simulink model "PV_model"  (R2018b)
settings: Solver=ode15s  StartTime=0.0  StopTime=6300  MaxStep=0.4  RelTol=1e-3  EnableMultiTasking=on
InitFcn:
  | load model_data
StopFcn:
  | %Title: System Identification for a HVAC Model
  | %Authors: Harsha Mathur and Nassim Khaled
  | %Last Modified: 4/11/2019
  | 
  | %% Plotting Settings
  | set(0,'DefaultLineLineWidth',2)
  | set(0,'DefaultAxesFontWeight','bold')
  | set(0,'DefaultAxesFontName','Arial')
  | set(0,'DefaultAxesFontSize',12)
  | 
  | figure
  | subplot(2,1,1)
  | 
  | plot(Time_sim,Voltage_PV1_measured)
  | hold on
  | plot(Time_sim,Voltage_PV1_sim,'r')
  | title('PV 1')
  | legend('Measured','simulated')
  | ylabel('Voltage [V]')
  | ylim([0 15])
  | grid on
  | 
  | subplot(2,1,2)
  | plot(Time_sim,Power_PV1_measured)
  | hold on
  | plot(Time_sim,Power_PV1_sim,'r')
  | legend('Measured','simulated')
  | ylabel('Power [Watts]')
  | ylim([0 100])
  | grid on
  | xlabel('Time [sec]')
  | 
  | 
  | figure
  | subplot(2,1,1)
  | 
  | plot(Time_sim,Voltage_PV23_measured)
  | hold on
  | plot(Time_sim,Voltage_PV23_sim,'r')
  | title('PV 2 and 3')
  | legend('Measured','simulated')
  | ylabel('Voltage [V]')
  | ylim([0 15])
  | grid on
  | 
  | subplot(2,1,2)
  | plot(Time_sim,Power_PV23_measured)
  | hold on
  | plot(Time_sim,Power_PV23_sim,'r')
  | legend('Measured','simulated')
  | ylabel('Power [Watts]')
  | ylim([0 100])
  | grid on
  | xlabel('Time [sec]')
undefined symbols (not defined in the file or in its folder): C1_LUT, Capacity_LUT, cell_Cp_heat, cell_mass, Em_LUT, Qe_init, R0_LUT, R1_LUT, SOC_LUT, T_init, Temperature_LUT
libraries: elec_lib x117, fl_lib x36, LiBatteryElements_lib x12, nesl_utility x12
settings Model: Creator=Sanjay Lodwal  LastModifiedBy=user
settings DataIOCC: LimitDataPoints=on  SaveFormat=Array
settings OptimizationCC: LifeSpan=inf
settings DebuggingCC: UnderspecifiedInitializationDetection=Classic  MergeDetectMultiDrivingBlocksExec=none  SolverPrmCheckMsg=warning  StateNameClashWarn=warning  SFUnexpectedBacktrackingDiag=warning  SFNoUnconditionalDefaultTransitionDiag=warning  SFExecutionAtInitializationDiag=none
settings HardwareCC: ProdBitPerPointer=32  ProdBitPerSizeT=32  ProdBitPerPtrDiffT=32  ProdLargestAtomicFloat=None  ProdIntDivRoundTo=Undefined  ProdEndianess=Unspecified  ProdWordSize=32  ProdHWDeviceType=32-bit Generic
settings ModelReferenceCC: PropagateSignalLabelsOutOfModel=off
settings SFSimCC: SimUseLocalCustomCode=off
settings RTWCC: RTWUseLocalCustomCode=off
settings CodeAppCC: StateflowObjectComments=on
settings GRTTargetCC: TargetLangStandard=C89/C90 (ANSI)  GeneratePreprocessorConditionals=Disable all
settings ConfigComp: CovMetricSettings=dw  CovHtmlReporting=on  CovSaveCumulativeToWorkspaceVar=on  CovSaveSingleToWorkspaceVar=on  CovExternalEMLEnable=off
settings SimscapeCC: SimscapeNormalizeSystem=off

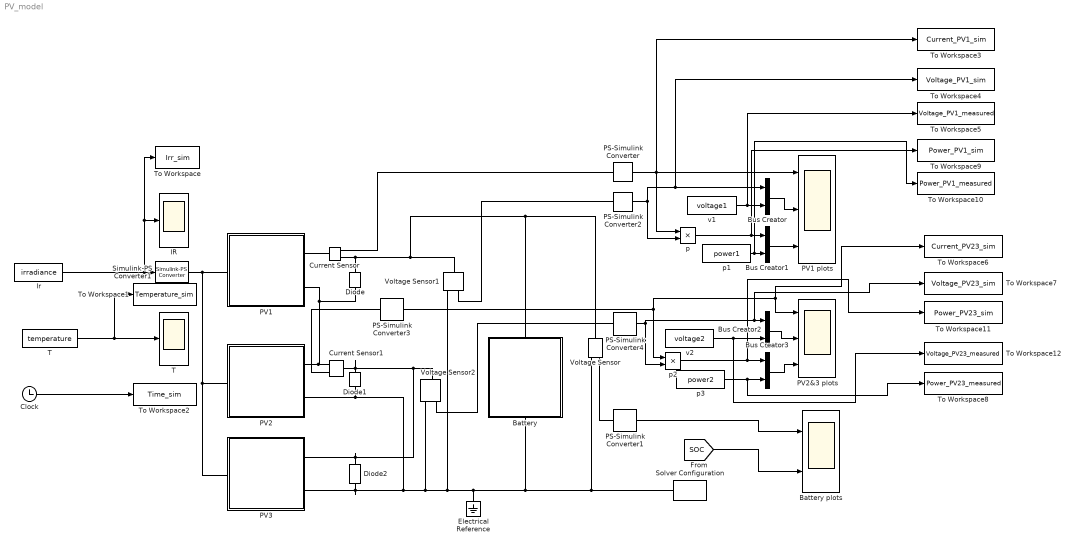
== system PV_model ==
  "\tT" : Scope
  Battery : Subsystem
      mask Display: image('battery.png')
  Battery plots : Scope  NumInputPorts=2
  Bus Creator{,1..3} (4 alike) : BusCreator  Inputs=2
  Clock : Clock
  Current Sensor : fl_lib/Electrical/Electrical Sensors/Current Sensor
  Current Sensor1 : fl_lib/Electrical/Electrical Sensors/Current Sensor
  Diode : fl_lib/Electrical/Electrical Elements/Diode  Vf=0.6 V  Ron=0.3 Ohm  Goff=1e-8 1/Ohm  i_specify=off  i_priority=High  i=0 A  i_nominal_specify=off  i_nominal_unit=A  i_nominal_value=1  v_specify=off  v_priority=High  v=0 V  v_nominal_specify=off  v_nominal_unit=V  v_nominal_value=1
  Diode1 : fl_lib/Electrical/Electrical Elements/Diode  Vf=0.6 V  Ron=0.3 Ohm  Goff=1e-8 1/Ohm  i_specify=off  i_priority=High  i=0 A  i_nominal_specify=off  i_nominal_unit=A  i_nominal_value=1  v_specify=off  v_priority=High  v=0 V  v_nominal_specify=off  v_nominal_unit=V  v_nominal_value=1
  Diode2 : fl_lib/Electrical/Electrical Elements/Diode  Vf=0.6 V  Ron=0.3 Ohm  Goff=1e-8 1/Ohm  i_specify=off  i_priority=High  i=0 A  i_nominal_specify=off  i_nominal_unit=A  i_nominal_value=1  v_specify=off  v_priority=High  v=0 V  v_nominal_specify=off  v_nominal_unit=V  v_nominal_value=1
  Electrical Reference : fl_lib/Electrical/Electrical Elements/Electrical Reference
  IR : Scope
  Ir : FromWorkspace  VariableName=irradiance  SampleTime=0
  PS-Simulink Converter{,1..4} (5 alike) : nesl_utility/PS-Simulink Converter  PhysicalDomain=network_engine_domain  SubClassName=ps_output  LeftPortType=input  RightPortType=output  PseudoPeriodic=off  Frequencies=[]  Unit=1  AffineConversion=off
  PV1 : Subsystem  mask{Isc=5.49, Voc=21.5, n=1.5, Rs=0, Ir0=1000, T=30}
      mask prompts: Isc "Short circuit current"; Voc "Open circuit voltage"; n "Quality factor, N"; Rs "Series resistance"; Ir0 "Reference irradiation"; T "Temperature"
      mask Display: image('PV1.jpg')
  PV1 plots : Scope  NumInputPorts=3
  PV2 : Subsystem  mask{Isc=6.37, Voc=21.5, n=1.5, Rs=0, Ir0=1000, T=30}
      mask prompts: Isc "Short circuit current"; Voc "Open circuit voltage"; n "Quality factor, N"; Rs "Series resistance"; Ir0 "Reference irradiation"; T "Temperature"
      mask Display: image('PV2.jpg')
  PV2&3 plots : Scope  NumInputPorts=3
  PV3 : Subsystem  mask{Isc=6.37, Voc=21.5, n=1.5, Rs=0, Ir0=1000, T=30}
      mask prompts: Isc "Short circuit current"; Voc "Open circuit voltage"; n "Quality factor, N"; Rs "Series resistance"; Ir0 "Reference irradiation"; T "Temperature"
      mask Display: image('PV3.jpg')
  Simulink-PS Converter1 : nesl_utility/Simulink-PS Converter  PhysicalDomain=network_engine_domain  SubClassName=ps_input  LeftPortType=input  RightPortType=output  PseudoPeriodic=off  Frequencies=[]  NoiseDistribution=none  NoiseParameters=[]  Unit=1  AffineConversion=off  FilteringAndDerivatives=zero  SimscapeFilterOrder=1  InputFilterTimeConstant=0.001  UdotUserProvided=1
  Solver Configuration : nesl_utility/Solver Configuration  PhysicalDomain=network_engine_domain  SubClassName=solver  LeftPortType=input  RightPortType=generic  Tones=[]  Harmonics=[]  SimulateNoise=off  Profile=off  UseLocalSampling=off  EnableSwitchedLinearOptims=on  FrequencyDomain=off  UseCCode=off  RelTol=0.001  AbsTol=1e-06  MinStep=1e-09  ToWorkspace=off  RevertToSquareIcSolve=off  NumHomotopyIterations=100  PhasorMode=off  PhasorModeNumHarmonics=1  DoDC=off  ResidualTolerance=1e-09  UseLocalSolver=off  LocalSolverChoice=NE_BACKWARD_EULER_ADVANCER  LocalSolverSampleTime=0.001  DoFixedCost=off  MaxNonlinIter=3  MaxModeIter=2  LinearAlgebra=Sparse  EquationFormulation=NE_TIME_EF  DelaysMemoryBudget=1024  AutomaticFiltering=on  FilteringTimeConstant=0.001  PartitionStorageMethod=AS_NEEDED  PartitionMemoryBudget=1024
  T : FromWorkspace  VariableName=temperature  SampleTime=0
  To Workspace : ToWorkspace  VariableName=Irr_sim  SampleTime=-1
  To Workspace1 : ToWorkspace  VariableName=Temperature_sim  SampleTime=-1
  To Workspace10 : ToWorkspace  VariableName=Power_PV1_measured  SampleTime=-1
  To Workspace11 : ToWorkspace  VariableName=Power_PV23_sim  SampleTime=-1
  To Workspace12 : ToWorkspace  VariableName=Voltage_PV23_measured  SampleTime=-1
  To Workspace2 : ToWorkspace  VariableName=Time_sim  SampleTime=-1
  To Workspace3 : ToWorkspace  VariableName=Current_PV1_sim  SampleTime=-1
  To Workspace4 : ToWorkspace  VariableName=Voltage_PV1_sim  SampleTime=-1
  To Workspace5 : ToWorkspace  VariableName=Voltage_PV1_measured  SampleTime=-1
  To Workspace6 : ToWorkspace  VariableName=Current_PV23_sim  SampleTime=-1
  To Workspace7 : ToWorkspace  VariableName=Voltage_PV23_sim  SampleTime=-1
  To Workspace8 : ToWorkspace  VariableName=Power_PV23_measured  SampleTime=-1
  To Workspace9 : ToWorkspace  VariableName=Power_PV1_sim  SampleTime=-1
  Voltage Sensor : fl_lib/Electrical/Electrical Sensors/Voltage Sensor
  Voltage Sensor1 : fl_lib/Electrical/Electrical Sensors/Voltage Sensor
  Voltage Sensor2 : fl_lib/Electrical/Electrical Sensors/Voltage Sensor
  p : Product
  p1 : FromWorkspace  VariableName=power1  SampleTime=0
  p2 : Product
  p3 : FromWorkspace  VariableName=power2  SampleTime=0
  v1 : FromWorkspace  VariableName=voltage1  SampleTime=0
  v2 : FromWorkspace  VariableName=voltage2  SampleTime=0
  wires:
  Ir/1 -> To Workspace/1, IR/1, Simulink-PS Converter1/1
  PS-Simulink Converter/1 -> To Workspace3/1, PV1 plots/1, p/1
  PS-Simulink Converter2/1 -> To Workspace4/1, Bus Creator/1, p/2
  PS-Simulink Converter4/1 -> p2/2, To Workspace7/1, Bus Creator2/1
  [SOC] -> Battery plots/2
  PS-Simulink Converter1/1 -> Battery plots/1
  T/1 -> To Workspace1/1, "\tT"/1
  v1/1 -> To Workspace5/1, Bus Creator/2
  Bus Creator/1 -> PV1 plots/2
  Bus Creator1/1 -> PV1 plots/3
  p/1 -> To Workspace9/1, Bus Creator1/1
  p1/1 -> To Workspace10/1, Bus Creator1/2
  PS-Simulink Converter3/1 -> To Workspace6/1, PV2&3 plots/1, p2/1
  Bus Creator2/1 -> PV2&3 plots/2
  v2/1 -> To Workspace12/1, Bus Creator2/2
  p2/1 -> To Workspace11/1, Bus Creator3/1
  p3/1 -> To Workspace8/1, Bus Creator3/2
  Bus Creator3/1 -> PV2&3 plots/3
  Clock/1 -> To Workspace2/1
  connections:
  Simulink-PS Converter1/RConn1 -- PV3/LConn1 -- PV2/LConn1 -- PV1/LConn1
  Current Sensor/RConn1 -- PS-Simulink Converter/LConn1
  PS-Simulink Converter1/LConn1 -- Voltage Sensor/RConn1
  Battery/RConn1 -- Voltage Sensor/LConn1 -- Voltage Sensor1/LConn1 -- Diode/RConn1 -- Current Sensor/RConn2
  Diode1/RConn1 -- Current Sensor1/LConn1 -- Voltage Sensor2/LConn1 -- PV3/RConn1 -- Diode2/RConn1
  PS-Simulink Converter2/LConn1 -- Voltage Sensor1/RConn1
  PS-Simulink Converter3/LConn1 -- Current Sensor1/RConn1
  PS-Simulink Converter4/LConn1 -- Voltage Sensor2/RConn1
  Solver Configuration/RConn1 -- Battery/LConn1 -- Electrical Reference/LConn1 -- Voltage Sensor1/RConn2 -- PV3/RConn2 -- Diode2/LConn1 -- PV2/RConn2 -- Diode1/LConn1 -- Voltage Sensor2/RConn2 -- Voltage Sensor/RConn2
  Current Sensor/LConn1 -- PV1/RConn1
  PV2/RConn1 -- Diode/LConn1 -- PV1/RConn2 -- Current Sensor1/RConn2

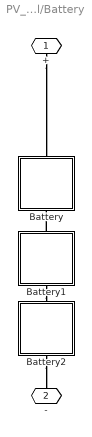
== system PV_model/Battery ==
  Battery : Subsystem  mask(Lithium cell (one RC-branch equivalent circuit)){Qe_init=Qe_init, T_init=T_init, Capacity_LUT=Capacity_LUT, Em_LUT=Em_LUT, R0_LUT=R0_LUT, R1_LUT=R1_LUT, C1_LUT=C1_LUT, cell_mass=cell_mass, cell_Cp_heat=cell_Cp_heat, SOC_LUT=SOC_LUT, Temperature_LUT=Temperature_LUT}
      mask prompts: Qe_init "Initial charge deficit (A*hr)"; T_init "Initial cell temperature (K)"; Capacity_LUT "Capacity (A*hr, 1xN table)"; Em_LUT "Em open-circuit voltage (volts, MxN table)"; R0_LUT "R0 terminal resistance (ohms, MxN table)"; R1_LUT "R1 resistance (ohms, MxN table)"; C1_LUT "C1 capacitance (farads, MxN table)"; cell_mass "Cell mass (kg)"; cell_Cp_heat "Cell specific heat (J/kg/K)"; SOC_LUT "SOC table breakpoints (Mx1 array)"; Temperature_LUT "Temperature table breakpoints (K, 1xN array)"
      mask DialogControl ParameterTabVar0 Prompt: Initial Conditions
      mask DialogControl ParameterTabVar01 Prompt: Electrical
      mask DialogControl ParameterTabVar012 Prompt: Thermal
      mask DialogControl ParameterTabVar0123 Prompt: Table Breakpoints
      mask Display:
      | image('battery.jpg')
      | color('red')
      | port_label('LConn',1,'H')
      | port_label('LConn',2,'+')
      | port_label('RConn',1,'-')
  Battery1 : Subsystem  mask(Lithium cell (one RC-branch equivalent circuit)){Qe_init=Qe_init, T_init=T_init, Capacity_LUT=Capacity_LUT, Em_LUT=Em_LUT, R0_LUT=R0_LUT, R1_LUT=R1_LUT, C1_LUT=C1_LUT, cell_mass=cell_mass, cell_Cp_heat=cell_Cp_heat, SOC_LUT=SOC_LUT, Temperature_LUT=Temperature_LUT}
      mask prompts: Qe_init "Initial charge deficit (A*hr)"; T_init "Initial cell temperature (K)"; Capacity_LUT "Capacity (A*hr, 1xN table)"; Em_LUT "Em open-circuit voltage (volts, MxN table)"; R0_LUT "R0 terminal resistance (ohms, MxN table)"; R1_LUT "R1 resistance (ohms, MxN table)"; C1_LUT "C1 capacitance (farads, MxN table)"; cell_mass "Cell mass (kg)"; cell_Cp_heat "Cell specific heat (J/kg/K)"; SOC_LUT "SOC table breakpoints (Mx1 array)"; Temperature_LUT "Temperature table breakpoints (K, 1xN array)"
      mask DialogControl ParameterTabVar0 Prompt: Initial Conditions
      mask DialogControl ParameterTabVar01 Prompt: Electrical
      mask DialogControl ParameterTabVar012 Prompt: Thermal
      mask DialogControl ParameterTabVar0123 Prompt: Table Breakpoints
      mask Display:
      | image('battery.jpg')
      | color('red')
      | port_label('LConn',1,'H')
      | port_label('LConn',2,'+')
      | port_label('RConn',1,'-')
  Battery2 : Subsystem  mask(Lithium cell (one RC-branch equivalent circuit)){Qe_init=Qe_init, T_init=T_init, Capacity_LUT=Capacity_LUT, Em_LUT=Em_LUT, R0_LUT=R0_LUT, R1_LUT=R1_LUT, C1_LUT=C1_LUT, cell_mass=cell_mass, cell_Cp_heat=cell_Cp_heat, SOC_LUT=SOC_LUT, Temperature_LUT=Temperature_LUT}
      mask prompts: Qe_init "Initial charge deficit (A*hr)"; T_init "Initial cell temperature (K)"; Capacity_LUT "Capacity (A*hr, 1xN table)"; Em_LUT "Em open-circuit voltage (volts, MxN table)"; R0_LUT "R0 terminal resistance (ohms, MxN table)"; R1_LUT "R1 resistance (ohms, MxN table)"; C1_LUT "C1 capacitance (farads, MxN table)"; cell_mass "Cell mass (kg)"; cell_Cp_heat "Cell specific heat (J/kg/K)"; SOC_LUT "SOC table breakpoints (Mx1 array)"; Temperature_LUT "Temperature table breakpoints (K, 1xN array)"
      mask DialogControl ParameterTabVar0 Prompt: Initial Conditions
      mask DialogControl ParameterTabVar01 Prompt: Electrical
      mask DialogControl ParameterTabVar012 Prompt: Thermal
      mask DialogControl ParameterTabVar0123 Prompt: Table Breakpoints
      mask Display:
      | image('battery.jpg')
      | color('red')
      | port_label('LConn',1,'H')
      | port_label('LConn',2,'+')
      | port_label('RConn',1,'-')
  + : PMIOPort  Side=Right
  - : PMIOPort  Port=2  Side=Left
  connections:
  +/RConn1 -- Battery/LConn1
  Battery1/LConn1 -- Battery/RConn1
  Battery1/RConn1 -- Battery2/LConn1
  Battery2/RConn1 -- -/RConn1

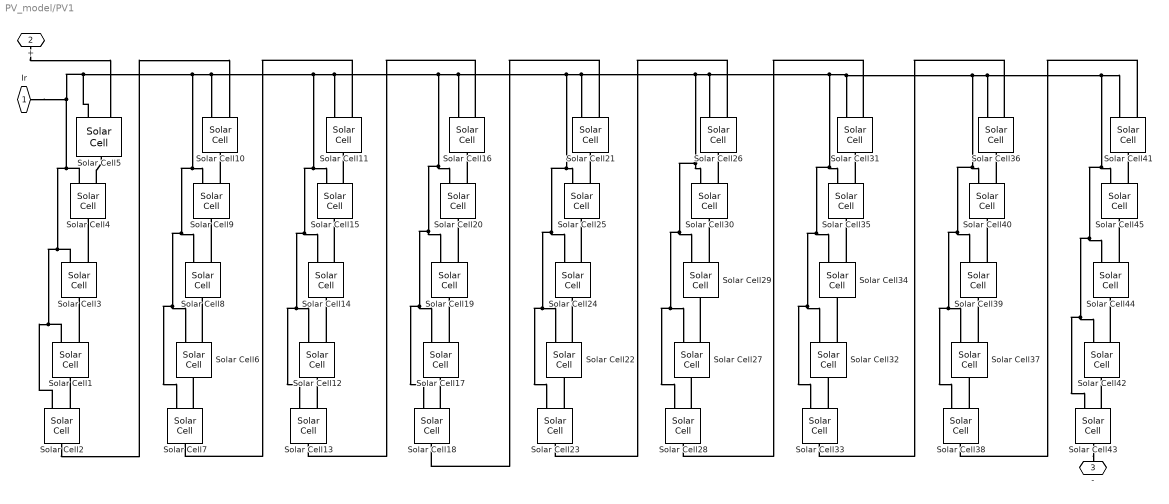
== system PV_model/PV1 ==
  Solar Cell{1..45} (45 alike) : elec_lib/Sources/Solar Cell  prm=1  Isc=Isc A  Voc=Voc/45 V  Is=1e-6 A  Is2=0 A  Iph=7.34 A  Ir0=Ir0 W/m^2  ec=n  N2=2  Rs=Rs/45 Ohm  Rp=Inf Ohm  N_series=1  TIPH1=0 1/K  EG=1.11 eV  TXIS1=3  TXIS2=3  TRS1=0  TRP1=0  Tmeas=T degC  TFIXED=T degC  thermal_mass=100 J/K  initial_temperature=25 degC
      settings: SourceProductName=Simscape Electronics  SourceProductBaseCode=SN
  Ir : PMIOPort  Side=Left
  + : PMIOPort  Port=2  Side=Right
  - : PMIOPort  Port=3  Side=Right
  connections:
  Solar Cell5/LConn1 -- Solar Cell7/LConn1 -- Solar Cell6/LConn1 -- Solar Cell8/LConn1 -- Solar Cell9/LConn1 -- Solar Cell13/LConn1 -- Solar Cell12/LConn1 -- Solar Cell14/LConn1 -- Solar Cell15/LConn1 -- Solar Cell18/LConn1 -- Solar Cell17/LConn1 -- Solar Cell19/LConn1 -- Solar Cell20/LConn1 -- Solar Cell22/LConn1 -- Solar Cell23/LConn1 -- Solar Cell24/LConn1 -- Solar Cell25/LConn1 -- Solar Cell28/LConn1 -- Solar Cell27/LConn1 -- Solar Cell29/LConn1 -- Solar Cell30/LConn1 -- Solar Cell33/LConn1 -- Solar Cell32/LConn1 -- Solar Cell34/LConn1 -- Solar Cell35/LConn1 -- Solar Cell37/LConn1 -- Solar Cell38/LConn1 -- Solar Cell39/LConn1 -- Solar Cell40/LConn1 -- Solar Cell43/LConn1 -- Solar Cell42/LConn1 -- Solar Cell44/LConn1 -- Solar Cell45/LConn1 -- Solar Cell41/LConn1 -- Solar Cell36/LConn1 -- Solar Cell31/LConn1 -- Solar Cell26/LConn1 -- Solar Cell21/LConn1 -- Solar Cell16/LConn1 -- Solar Cell11/LConn1 -- Solar Cell10/LConn1 -- Solar Cell4/LConn1 -- Solar Cell3/LConn1 -- Solar Cell1/LConn1 -- Solar Cell2/LConn1 -- Ir/RConn1
  Solar Cell3/LConn2 -- Solar Cell4/RConn1
  Solar Cell2/LConn2 -- Solar Cell1/RConn1
  Solar Cell1/LConn2 -- Solar Cell3/RConn1
  Solar Cell4/LConn2 -- Solar Cell5/RConn1
  +/RConn1 -- Solar Cell5/LConn2
  Solar Cell9/LConn2 -- Solar Cell10/RConn1
  Solar Cell7/LConn2 -- Solar Cell6/RConn1
  Solar Cell6/LConn2 -- Solar Cell8/RConn1
  Solar Cell2/RConn1 -- Solar Cell10/LConn2
  Solar Cell8/LConn2 -- Solar Cell9/RConn1
  Solar Cell11/LConn2 -- Solar Cell7/RConn1
  Solar Cell12/LConn2 -- Solar Cell14/RConn1
  Solar Cell13/LConn2 -- Solar Cell12/RConn1
  Solar Cell15/LConn2 -- Solar Cell11/RConn1
  Solar Cell14/LConn2 -- Solar Cell15/RConn1
  Solar Cell19/LConn2 -- Solar Cell20/RConn1
  Solar Cell20/LConn2 -- Solar Cell16/RConn1
  Solar Cell16/LConn2 -- Solar Cell13/RConn1
  Solar Cell17/LConn2 -- Solar Cell19/RConn1
  Solar Cell18/LConn2 -- Solar Cell17/RConn1
  Solar Cell23/LConn2 -- Solar Cell22/RConn1
  Solar Cell22/LConn2 -- Solar Cell24/RConn1
  Solar Cell25/LConn2 -- Solar Cell21/RConn1
  Solar Cell21/LConn2 -- Solar Cell18/RConn1
  Solar Cell24/LConn2 -- Solar Cell25/RConn1
  Solar Cell29/LConn2 -- Solar Cell30/RConn1
  Solar Cell26/LConn2 -- Solar Cell23/RConn1
  Solar Cell30/LConn2 -- Solar Cell26/RConn1
  Solar Cell27/LConn2 -- Solar Cell29/RConn1
  Solar Cell28/LConn2 -- Solar Cell27/RConn1
  Solar Cell34/LConn2 -- Solar Cell35/RConn1
  Solar Cell31/LConn2 -- Solar Cell28/RConn1
  Solar Cell35/LConn2 -- Solar Cell31/RConn1
  Solar Cell32/LConn2 -- Solar Cell34/RConn1
  Solar Cell33/LConn2 -- Solar Cell32/RConn1
  Solar Cell39/LConn2 -- Solar Cell40/RConn1
  Solar Cell36/LConn2 -- Solar Cell33/RConn1
  Solar Cell40/LConn2 -- Solar Cell36/RConn1
  Solar Cell37/LConn2 -- Solar Cell39/RConn1
  Solar Cell38/LConn2 -- Solar Cell37/RConn1
  Solar Cell44/LConn2 -- Solar Cell45/RConn1
  Solar Cell41/LConn2 -- Solar Cell38/RConn1
  Solar Cell45/LConn2 -- Solar Cell41/RConn1
  Solar Cell42/LConn2 -- Solar Cell44/RConn1
  Solar Cell43/LConn2 -- Solar Cell42/RConn1
  Solar Cell43/RConn1 -- -/RConn1

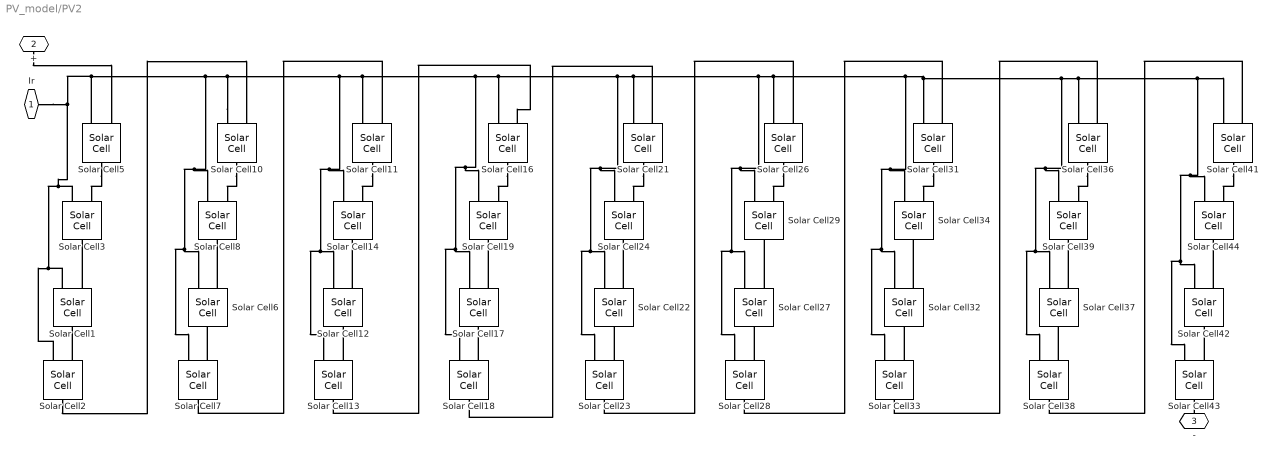
== system PV_model/PV2 ==
  Solar Cell{1..3,5..8,10..14,16..19,21..24,26..29,31..34,36..39,41..44} (36 alike) : elec_lib/Sources/Solar Cell  prm=1  Isc=Isc A  Voc=Voc/45 V  Is=1e-6 A  Is2=0 A  Iph=7.34 A  Ir0=Ir0 W/m^2  ec=n  N2=2  Rs=Rs/45 Ohm  Rp=Inf Ohm  N_series=1  TIPH1=0 1/K  EG=1.11 eV  TXIS1=3  TXIS2=3  TRS1=0  TRP1=0  Tmeas=T degC  TFIXED=T degC  thermal_mass=100 J/K  initial_temperature=25 degC
      settings: SourceProductName=Simscape Electronics  SourceProductBaseCode=SN
  Ir : PMIOPort  Side=Left
  + : PMIOPort  Port=2  Side=Right
  - : PMIOPort  Port=3  Side=Right
  connections:
  Solar Cell10/LConn1 -- Solar Cell13/LConn1 -- Solar Cell12/LConn1 -- Solar Cell14/LConn1 -- Solar Cell18/LConn1 -- Solar Cell17/LConn1 -- Solar Cell19/LConn1 -- Solar Cell22/LConn1 -- Solar Cell23/LConn1 -- Solar Cell24/LConn1 -- Solar Cell28/LConn1 -- Solar Cell27/LConn1 -- Solar Cell29/LConn1 -- Solar Cell33/LConn1 -- Solar Cell32/LConn1 -- Solar Cell34/LConn1 -- Solar Cell37/LConn1 -- Solar Cell38/LConn1 -- Solar Cell39/LConn1 -- Solar Cell41/LConn1 -- Solar Cell43/LConn1 -- Solar Cell42/LConn1 -- Solar Cell44/LConn1 -- Solar Cell36/LConn1 -- Solar Cell31/LConn1 -- Solar Cell26/LConn1 -- Solar Cell21/LConn1 -- Solar Cell16/LConn1 -- Solar Cell11/LConn1 -- Solar Cell5/LConn1 -- Ir/RConn1 -- Solar Cell3/LConn1 -- Solar Cell1/LConn1 -- Solar Cell2/LConn1 -- Solar Cell8/LConn1 -- Solar Cell7/LConn1 -- Solar Cell6/LConn1
  Solar Cell10/RConn1 -- Solar Cell8/LConn2
  Solar Cell1/LConn2 -- Solar Cell3/RConn1
  Solar Cell38/LConn2 -- Solar Cell37/RConn1
  Solar Cell18/LConn2 -- Solar Cell17/RConn1
  Solar Cell7/LConn2 -- Solar Cell6/RConn1
  Solar Cell21/LConn2 -- Solar Cell18/RConn1
  Solar Cell11/RConn1 -- Solar Cell14/LConn2
  Solar Cell31/LConn2 -- Solar Cell28/RConn1
  Solar Cell13/LConn2 -- Solar Cell12/RConn1
  Solar Cell32/LConn2 -- Solar Cell34/RConn1
  Solar Cell22/LConn2 -- Solar Cell24/RConn1
  Solar Cell23/LConn2 -- Solar Cell22/RConn1
  Solar Cell36/LConn2 -- Solar Cell33/RConn1
  Solar Cell2/LConn2 -- Solar Cell1/RConn1
  Solar Cell41/LConn2 -- Solar Cell38/RConn1
  Solar Cell27/LConn2 -- Solar Cell29/RConn1
  Solar Cell12/LConn2 -- Solar Cell14/RConn1
  Solar Cell16/RConn1 -- Solar Cell19/LConn2
  +/RConn1 -- Solar Cell5/LConn2
  Solar Cell28/LConn2 -- Solar Cell27/RConn1
  Solar Cell16/LConn2 -- Solar Cell13/RConn1
  Solar Cell43/LConn2 -- Solar Cell42/RConn1
  Solar Cell33/LConn2 -- Solar Cell32/RConn1
  Solar Cell41/RConn1 -- Solar Cell44/LConn2
  Solar Cell6/LConn2 -- Solar Cell8/RConn1
  Solar Cell2/RConn1 -- Solar Cell10/LConn2
  Solar Cell17/LConn2 -- Solar Cell19/RConn1
  -/RConn1 -- Solar Cell43/RConn1
  Solar Cell11/LConn2 -- Solar Cell7/RConn1
  Solar Cell26/LConn2 -- Solar Cell23/RConn1
  Solar Cell42/LConn2 -- Solar Cell44/RConn1
  Solar Cell37/LConn2 -- Solar Cell39/RConn1
  Solar Cell5/RConn1 -- Solar Cell3/LConn2
  Solar Cell21/RConn1 -- Solar Cell24/LConn2
  Solar Cell26/RConn1 -- Solar Cell29/LConn2
  Solar Cell31/RConn1 -- Solar Cell34/LConn2
  Solar Cell36/RConn1 -- Solar Cell39/LConn2

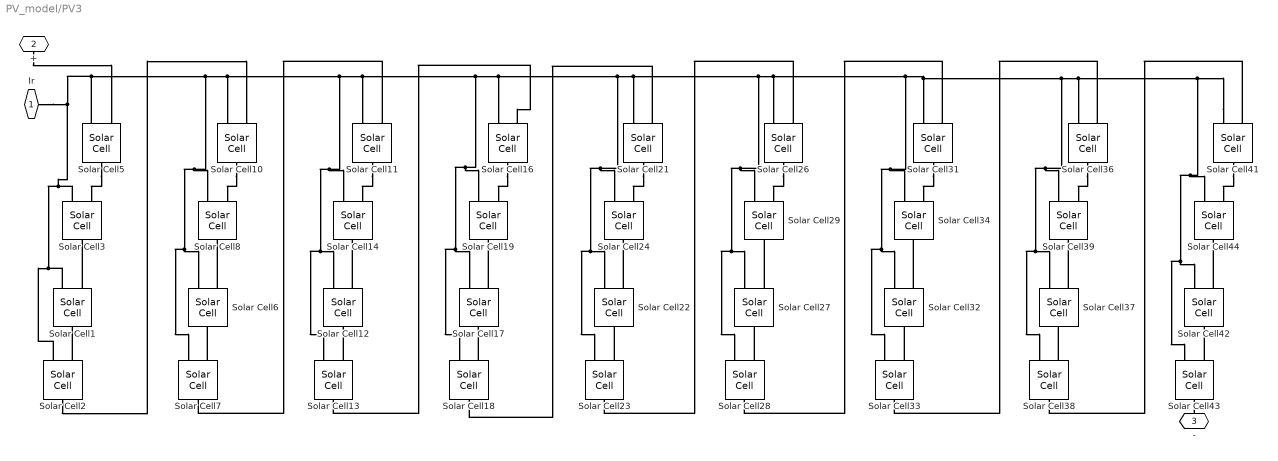
== system PV_model/PV3 ==
  Solar Cell{1..3,5..8,10..14,16..19,21..24,26..29,31..34,36..39,41..44} (36 alike) : elec_lib/Sources/Solar Cell  prm=1  Isc=Isc A  Voc=Voc/45 V  Is=1e-6 A  Is2=0 A  Iph=7.34 A  Ir0=Ir0 W/m^2  ec=n  N2=2  Rs=Rs/45 Ohm  Rp=Inf Ohm  N_series=1  TIPH1=0 1/K  EG=1.11 eV  TXIS1=3  TXIS2=3  TRS1=0  TRP1=0  Tmeas=T degC  TFIXED=T degC  thermal_mass=100 J/K  initial_temperature=25 degC
      settings: SourceProductName=Simscape Electronics  SourceProductBaseCode=SN
  Ir : PMIOPort  Side=Left
  + : PMIOPort  Port=2  Side=Right
  - : PMIOPort  Port=3  Side=Right
  connections:
  Solar Cell36/RConn1 -- Solar Cell39/LConn2
  Solar Cell31/RConn1 -- Solar Cell34/LConn2
  Solar Cell26/RConn1 -- Solar Cell29/LConn2
  Solar Cell21/RConn1 -- Solar Cell24/LConn2
  Solar Cell5/RConn1 -- Solar Cell3/LConn2
  Solar Cell37/LConn2 -- Solar Cell39/RConn1
  Solar Cell42/LConn2 -- Solar Cell44/RConn1
  Solar Cell26/LConn2 -- Solar Cell23/RConn1
  Solar Cell11/LConn2 -- Solar Cell7/RConn1
  -/RConn1 -- Solar Cell43/RConn1
  Solar Cell17/LConn2 -- Solar Cell19/RConn1
  Solar Cell2/RConn1 -- Solar Cell10/LConn2
  Solar Cell6/LConn2 -- Solar Cell8/RConn1
  Solar Cell41/RConn1 -- Solar Cell44/LConn2
  Solar Cell33/LConn2 -- Solar Cell32/RConn1
  Solar Cell43/LConn2 -- Solar Cell42/RConn1
  Solar Cell16/LConn2 -- Solar Cell13/RConn1
  Solar Cell28/LConn2 -- Solar Cell27/RConn1
  +/RConn1 -- Solar Cell5/LConn2
  Solar Cell16/RConn1 -- Solar Cell19/LConn2
  Solar Cell12/LConn2 -- Solar Cell14/RConn1
  Solar Cell27/LConn2 -- Solar Cell29/RConn1
  Solar Cell41/LConn2 -- Solar Cell38/RConn1
  Solar Cell2/LConn2 -- Solar Cell1/RConn1
  Solar Cell36/LConn2 -- Solar Cell33/RConn1
  Solar Cell23/LConn2 -- Solar Cell22/RConn1
  Solar Cell22/LConn2 -- Solar Cell24/RConn1
  Solar Cell32/LConn2 -- Solar Cell34/RConn1
  Solar Cell13/LConn2 -- Solar Cell12/RConn1
  Solar Cell31/LConn2 -- Solar Cell28/RConn1
  Solar Cell11/RConn1 -- Solar Cell14/LConn2
  Solar Cell21/LConn2 -- Solar Cell18/RConn1
  Solar Cell7/LConn2 -- Solar Cell6/RConn1
  Solar Cell18/LConn2 -- Solar Cell17/RConn1
  Solar Cell38/LConn2 -- Solar Cell37/RConn1
  Solar Cell1/LConn2 -- Solar Cell3/RConn1
  Solar Cell10/RConn1 -- Solar Cell8/LConn2
  Solar Cell41/LConn1 -- Solar Cell44/LConn1 -- Solar Cell42/LConn1 -- Solar Cell43/LConn1 -- Solar Cell6/LConn1 -- Solar Cell7/LConn1 -- Solar Cell8/LConn1 -- Solar Cell2/LConn1 -- Solar Cell1/LConn1 -- Solar Cell3/LConn1 -- Ir/RConn1 -- Solar Cell5/LConn1 -- Solar Cell10/LConn1 -- Solar Cell14/LConn1 -- Solar Cell12/LConn1 -- Solar Cell13/LConn1 -- Solar Cell11/LConn1 -- Solar Cell19/LConn1 -- Solar Cell17/LConn1 -- Solar Cell18/LConn1 -- Solar Cell16/LConn1 -- Solar Cell24/LConn1 -- Solar Cell23/LConn1 -- Solar Cell22/LConn1 -- Solar Cell21/LConn1 -- Solar Cell29/LConn1 -- Solar Cell27/LConn1 -- Solar Cell28/LConn1 -- Solar Cell26/LConn1 -- Solar Cell34/LConn1 -- Solar Cell32/LConn1 -- Solar Cell33/LConn1 -- Solar Cell31/LConn1 -- Solar Cell39/LConn1 -- Solar Cell38/LConn1 -- Solar Cell37/LConn1 -- Solar Cell36/LConn1

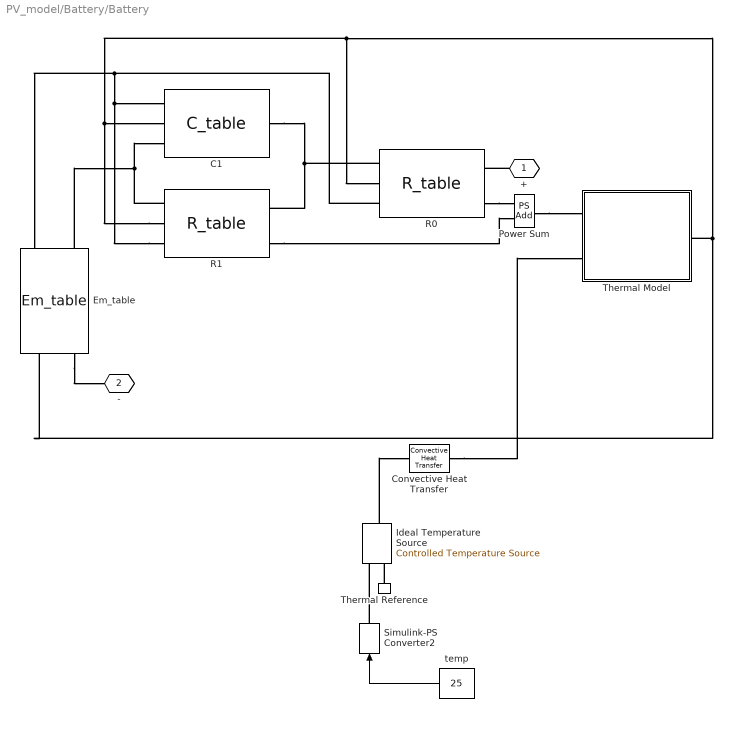
== system PV_model/Battery/Battery ==
  C1 : LiBatteryElements_lib/C_table  C_Table=C1_LUT F  SOC_Table=SOC_LUT  Temp_Table=Temperature_LUT K  v0=0 V
  Convective Heat Transfer : fl_lib/Thermal/Thermal Elements/Convective Heat Transfer  area=cell_area m^2  heat_tr_coeff=h_conv W/(m^2 * K)  T_specify=off  T_priority=High  T=0 K  T_nominal_specify=off  T_nominal_unit=K  T_nominal_value=1  Q_specify=off  Q_priority=High  Q=0 J/s  Q_nominal_specify=off  Q_nominal_unit=W  Q_nominal_value=1
  Em_table : LiBatteryElements_lib/Em_table  C_Table=Capacity_LUT hr*A  Em_Table=Em_LUT V  SOC_Table=SOC_LUT  Temp_Table=Temperature_LUT K  Qinit=Qe_init hr*A
  Ideal Temperature Source : fl_lib/Thermal/Thermal Sources/Controlled Temperature Source
      settings: SourceProductName=Simscape
  Power Sum : fl_lib/Physical Signals/Functions/PS Add
  R0 : LiBatteryElements_lib/R_table  R_Table=R0_LUT Ohm  SOC_Table=SOC_LUT  Temp_Table=Temperature_LUT K
  R1 : LiBatteryElements_lib/R_table  R_Table=R1_LUT Ohm  SOC_Table=SOC_LUT  Temp_Table=Temperature_LUT K
  Simulink-PS Converter2 : nesl_utility/Simulink-PS Converter  PhysicalDomain=network_engine_domain  SubClassName=ps_input  LeftPortType=input  RightPortType=output  PseudoPeriodic=off  Frequencies=[]  NoiseDistribution=none  NoiseParameters=[]  Unit=degC  AffineConversion=on  FilteringAndDerivatives=zero  SimscapeFilterOrder=1  InputFilterTimeConstant=.001  UdotUserProvided=1
  Thermal Model : Subsystem
  Thermal Reference : fl_lib/Thermal/Thermal Elements/Thermal Reference
  temp : Constant  Value=25
  + : PMIOPort  Tag=PMCPort  Side=Left
  - : PMIOPort  Tag=PMCPort  Port=2  Side=Right
  wires:
  temp/1 -> Simulink-PS Converter2/1
  connections:
  R1/LConn3 -- R0/LConn3 -- Em_table/LConn3 -- C1/LConn3
  Convective Heat Transfer/RConn1 -- Thermal Model/LConn2
  Em_table/RConn1 -- -/RConn1
  +/RConn1 -- R0/RConn1
  Em_table/LConn1 -- C1/LConn1 -- R1/LConn1
  R1/RConn2 -- Power Sum/LConn2
  R1/LConn2 -- Thermal Model/RConn1 -- Em_table/RConn2 -- R0/LConn2 -- C1/LConn2
  Power Sum/RConn1 -- Thermal Model/LConn1
  R1/RConn1 -- C1/RConn1 -- R0/LConn1
  R0/RConn2 -- Power Sum/LConn1
  Simulink-PS Converter2/RConn1 -- Ideal Temperature Source/RConn1
  Ideal Temperature Source/LConn1 -- Convective Heat Transfer/LConn1
  Thermal Reference/LConn1 -- Ideal Temperature Source/RConn2

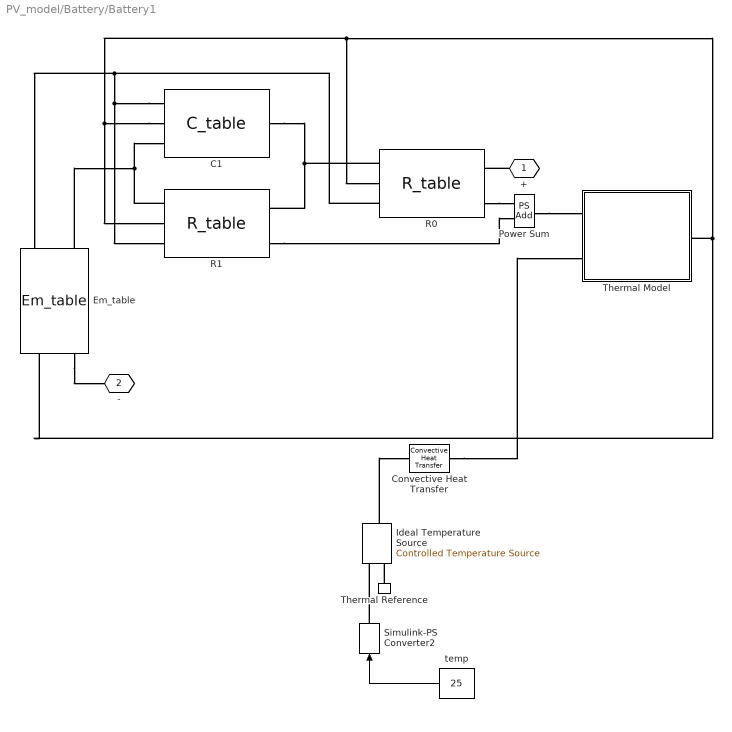
== system PV_model/Battery/Battery1 ==
  C1 : LiBatteryElements_lib/C_table  C_Table=C1_LUT F  SOC_Table=SOC_LUT  Temp_Table=Temperature_LUT K  v0=0 V
  Convective Heat Transfer : fl_lib/Thermal/Thermal Elements/Convective Heat Transfer  area=cell_area m^2  heat_tr_coeff=h_conv W/(m^2 * K)  T_specify=off  T_priority=High  T=0 K  T_nominal_specify=off  T_nominal_unit=K  T_nominal_value=1  Q_specify=off  Q_priority=High  Q=0 J/s  Q_nominal_specify=off  Q_nominal_unit=W  Q_nominal_value=1
  Em_table : LiBatteryElements_lib/Em_table  C_Table=Capacity_LUT hr*A  Em_Table=Em_LUT V  SOC_Table=SOC_LUT  Temp_Table=Temperature_LUT K  Qinit=Qe_init hr*A
  Ideal Temperature Source : fl_lib/Thermal/Thermal Sources/Controlled Temperature Source
      settings: SourceProductName=Simscape
  Power Sum : fl_lib/Physical Signals/Functions/PS Add
  R0 : LiBatteryElements_lib/R_table  R_Table=R0_LUT Ohm  SOC_Table=SOC_LUT  Temp_Table=Temperature_LUT K
  R1 : LiBatteryElements_lib/R_table  R_Table=R1_LUT Ohm  SOC_Table=SOC_LUT  Temp_Table=Temperature_LUT K
  Simulink-PS Converter2 : nesl_utility/Simulink-PS Converter  PhysicalDomain=network_engine_domain  SubClassName=ps_input  LeftPortType=input  RightPortType=output  PseudoPeriodic=off  Frequencies=[]  NoiseDistribution=none  NoiseParameters=[]  Unit=degC  AffineConversion=on  FilteringAndDerivatives=zero  SimscapeFilterOrder=1  InputFilterTimeConstant=.001  UdotUserProvided=1
  Thermal Model : Subsystem
  Thermal Reference : fl_lib/Thermal/Thermal Elements/Thermal Reference
  temp : Constant  Value=25
  + : PMIOPort  Tag=PMCPort  Side=Left
  - : PMIOPort  Tag=PMCPort  Port=2  Side=Right
  wires:
  temp/1 -> Simulink-PS Converter2/1
  connections:
  Thermal Reference/LConn1 -- Ideal Temperature Source/RConn2
  Ideal Temperature Source/LConn1 -- Convective Heat Transfer/LConn1
  Simulink-PS Converter2/RConn1 -- Ideal Temperature Source/RConn1
  R0/RConn2 -- Power Sum/LConn1
  R0/LConn1 -- C1/RConn1 -- R1/RConn1
  Power Sum/RConn1 -- Thermal Model/LConn1
  C1/LConn2 -- R0/LConn2 -- Em_table/RConn2 -- Thermal Model/RConn1 -- R1/LConn2
  R1/RConn2 -- Power Sum/LConn2
  R1/LConn1 -- C1/LConn1 -- Em_table/LConn1
  +/RConn1 -- R0/RConn1
  Em_table/RConn1 -- -/RConn1
  Convective Heat Transfer/RConn1 -- Thermal Model/LConn2
  C1/LConn3 -- R0/LConn3 -- Em_table/LConn3 -- R1/LConn3

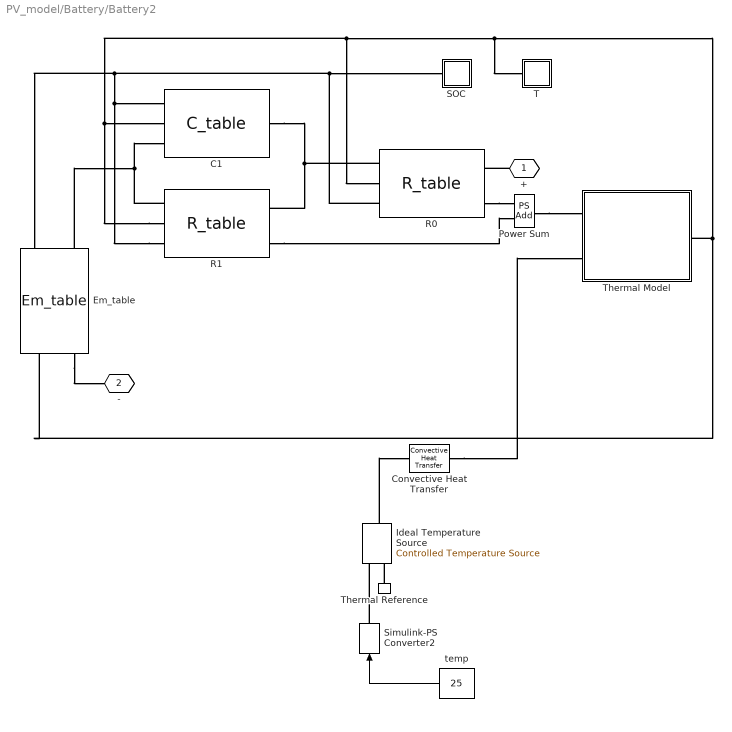
== system PV_model/Battery/Battery2 ==
  " SOC " : Subsystem
  C1 : LiBatteryElements_lib/C_table  C_Table=C1_LUT F  SOC_Table=SOC_LUT  Temp_Table=Temperature_LUT K  v0=0 V
  Convective Heat Transfer : fl_lib/Thermal/Thermal Elements/Convective Heat Transfer  area=cell_area m^2  heat_tr_coeff=h_conv W/(m^2 * K)  T_specify=off  T_priority=High  T=0 K  T_nominal_specify=off  T_nominal_unit=K  T_nominal_value=1  Q_specify=off  Q_priority=High  Q=0 J/s  Q_nominal_specify=off  Q_nominal_unit=W  Q_nominal_value=1
  Em_table : LiBatteryElements_lib/Em_table  C_Table=Capacity_LUT hr*A  Em_Table=Em_LUT V  SOC_Table=SOC_LUT  Temp_Table=Temperature_LUT K  Qinit=Qe_init hr*A
  Ideal Temperature Source : fl_lib/Thermal/Thermal Sources/Controlled Temperature Source
      settings: SourceProductName=Simscape
  Power Sum : fl_lib/Physical Signals/Functions/PS Add
  R0 : LiBatteryElements_lib/R_table  R_Table=R0_LUT Ohm  SOC_Table=SOC_LUT  Temp_Table=Temperature_LUT K
  R1 : LiBatteryElements_lib/R_table  R_Table=R1_LUT Ohm  SOC_Table=SOC_LUT  Temp_Table=Temperature_LUT K
  Simulink-PS Converter2 : nesl_utility/Simulink-PS Converter  PhysicalDomain=network_engine_domain  SubClassName=ps_input  LeftPortType=input  RightPortType=output  PseudoPeriodic=off  Frequencies=[]  NoiseDistribution=none  NoiseParameters=[]  Unit=degC  AffineConversion=on  FilteringAndDerivatives=zero  SimscapeFilterOrder=1  InputFilterTimeConstant=.001  UdotUserProvided=1
  T : Subsystem
  Thermal Model : Subsystem
  Thermal Reference : fl_lib/Thermal/Thermal Elements/Thermal Reference
  temp : Constant  Value=25
  + : PMIOPort  Tag=PMCPort  Side=Left
  - : PMIOPort  Tag=PMCPort  Port=2  Side=Right
  wires:
  temp/1 -> Simulink-PS Converter2/1
  connections:
  R1/LConn3 -- " SOC "/LConn1 -- R0/LConn3 -- Em_table/LConn3 -- C1/LConn3
  Convective Heat Transfer/RConn1 -- Thermal Model/LConn2
  Em_table/RConn1 -- -/RConn1
  +/RConn1 -- R0/RConn1
  Em_table/LConn1 -- C1/LConn1 -- R1/LConn1
  R1/RConn2 -- Power Sum/LConn2
  R1/LConn2 -- Thermal Model/RConn1 -- Em_table/RConn2 -- T/LConn1 -- R0/LConn2 -- C1/LConn2
  Power Sum/RConn1 -- Thermal Model/LConn1
  R1/RConn1 -- C1/RConn1 -- R0/LConn1
  R0/RConn2 -- Power Sum/LConn1
  Simulink-PS Converter2/RConn1 -- Ideal Temperature Source/RConn1
  Ideal Temperature Source/LConn1 -- Convective Heat Transfer/LConn1
  Thermal Reference/LConn1 -- Ideal Temperature Source/RConn2

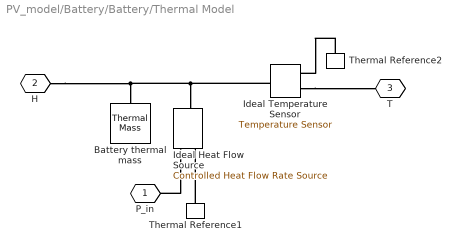
== system PV_model/Battery/Battery/Thermal Model ==
  Battery thermal mass : fl_lib/Thermal/Thermal Elements/Thermal Mass  mass=cell_mass kg  sp_heat=cell_Cp_heat J/kg/K  T_specify=on  T_priority=High  T=T_init K  T_nominal_specify=off  T_nominal_unit=K  T_nominal_value=1  Q_specify=off  Q_priority=High  Q=0 J/s  Q_nominal_specify=off  Q_nominal_unit=W  Q_nominal_value=1
  Ideal Temperature Sensor : fl_lib/Thermal/Thermal Sensors/Temperature Sensor
  Ideal Heat Flow Source : fl_lib/Thermal/Thermal Sources/Controlled Heat Flow Rate Source
      settings: SourceProductName=Simscape
  Thermal Reference1 : fl_lib/Thermal/Thermal Elements/Thermal Reference
  Thermal Reference2 : fl_lib/Thermal/Thermal Elements/Thermal Reference
  P_in : PMIOPort  Tag=PMCPort  Side=Left
  H : PMIOPort  Tag=PMCPort  Port=2  Side=Left
  T : PMIOPort  Tag=PMCPort  Port=3  Side=Right
  connections:
  Thermal Reference2/LConn1 -- Ideal Temperature Sensor/RConn1
  Ideal Temperature Sensor/RConn2 -- T/RConn1
  Thermal Reference1/LConn1 -- Ideal Heat Flow Source/RConn2
  Ideal Temperature Sensor/LConn1 -- H/RConn1 -- Battery thermal mass/LConn1 -- Ideal Heat Flow Source/LConn1
  Ideal Heat Flow Source/RConn1 -- P_in/RConn1

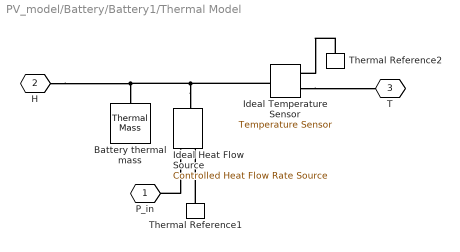
== system PV_model/Battery/Battery1/Thermal Model ==
  Battery thermal mass : fl_lib/Thermal/Thermal Elements/Thermal Mass  mass=cell_mass kg  sp_heat=cell_Cp_heat J/kg/K  T_specify=on  T_priority=High  T=T_init K  T_nominal_specify=off  T_nominal_unit=K  T_nominal_value=1  Q_specify=off  Q_priority=High  Q=0 J/s  Q_nominal_specify=off  Q_nominal_unit=W  Q_nominal_value=1
  Ideal Temperature Sensor : fl_lib/Thermal/Thermal Sensors/Temperature Sensor
  Ideal Heat Flow Source : fl_lib/Thermal/Thermal Sources/Controlled Heat Flow Rate Source
      settings: SourceProductName=Simscape
  Thermal Reference1 : fl_lib/Thermal/Thermal Elements/Thermal Reference
  Thermal Reference2 : fl_lib/Thermal/Thermal Elements/Thermal Reference
  P_in : PMIOPort  Tag=PMCPort  Side=Left
  H : PMIOPort  Tag=PMCPort  Port=2  Side=Left
  T : PMIOPort  Tag=PMCPort  Port=3  Side=Right
  connections:
  Ideal Heat Flow Source/RConn1 -- P_in/RConn1
  Ideal Heat Flow Source/LConn1 -- Battery thermal mass/LConn1 -- H/RConn1 -- Ideal Temperature Sensor/LConn1
  Thermal Reference1/LConn1 -- Ideal Heat Flow Source/RConn2
  Ideal Temperature Sensor/RConn2 -- T/RConn1
  Thermal Reference2/LConn1 -- Ideal Temperature Sensor/RConn1

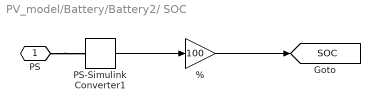
== system PV_model/Battery/Battery2/ SOC  ==
  % : Gain  Gain=100
  PS-Simulink Converter1 : nesl_utility/PS-Simulink Converter  PhysicalDomain=network_engine_domain  SubClassName=ps_output  LeftPortType=input  RightPortType=output  PseudoPeriodic=off  Frequencies=[]  Unit=1  AffineConversion=off
  PS : PMIOPort  Side=Left
  tag scope: SOC=global
  wires:
  PS-Simulink Converter1/1 -> %/1
  %/1 -> [SOC]
  connections:
  PS/RConn1 -- PS-Simulink Converter1/LConn1

== system PV_model/Battery/Battery2/T ==
  PS-Simulink Converter1 : nesl_utility/PS-Simulink Converter  PhysicalDomain=network_engine_domain  SubClassName=ps_output  LeftPortType=input  RightPortType=output  PseudoPeriodic=off  Frequencies=[]  Unit=degC  AffineConversion=on
  PS : PMIOPort  Side=Left
  tag scope: T=global
  wires:
  PS-Simulink Converter1/1 -> [T]
  connections:
  PS/RConn1 -- PS-Simulink Converter1/LConn1

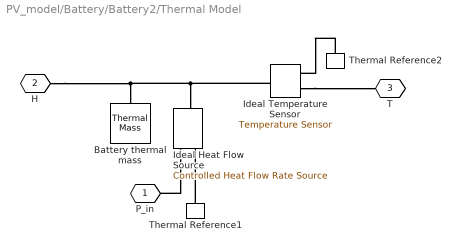
== system PV_model/Battery/Battery2/Thermal Model ==
  Battery thermal mass : fl_lib/Thermal/Thermal Elements/Thermal Mass  mass=cell_mass kg  sp_heat=cell_Cp_heat J/kg/K  T_specify=on  T_priority=High  T=T_init K  T_nominal_specify=off  T_nominal_unit=K  T_nominal_value=1  Q_specify=off  Q_priority=High  Q=0 J/s  Q_nominal_specify=off  Q_nominal_unit=W  Q_nominal_value=1
  Ideal Temperature Sensor : fl_lib/Thermal/Thermal Sensors/Temperature Sensor
  Ideal Heat Flow Source : fl_lib/Thermal/Thermal Sources/Controlled Heat Flow Rate Source
      settings: SourceProductName=Simscape
  Thermal Reference1 : fl_lib/Thermal/Thermal Elements/Thermal Reference
  Thermal Reference2 : fl_lib/Thermal/Thermal Elements/Thermal Reference
  P_in : PMIOPort  Tag=PMCPort  Side=Left
  H : PMIOPort  Tag=PMCPort  Port=2  Side=Left
  T : PMIOPort  Tag=PMCPort  Port=3  Side=Right
  connections:
  Thermal Reference2/LConn1 -- Ideal Temperature Sensor/RConn1
  Ideal Temperature Sensor/RConn2 -- T/RConn1
  Thermal Reference1/LConn1 -- Ideal Heat Flow Source/RConn2
  Ideal Temperature Sensor/LConn1 -- H/RConn1 -- Battery thermal mass/LConn1 -- Ideal Heat Flow Source/LConn1
  Ideal Heat Flow Source/RConn1 -- P_in/RConn1
